simulink model "PI_Controller"  (R2020b)
settings: Solver=VariableStepAuto  StartTime=0.0  StopTime=120  RelTol=1e-3
PostLoadFcn:
  | M=1000;
  | b=50;
  | u=500;
  | 
  | Kp=19.9969;
  | Ki=0.34998;
  | Ts=3.36;
InitFcn:
  | M=1000;
  | b=50;
  | u=500;
  | 
  | Kp=19.9969;
  | Ki=0.34998;
  | Ts=3.36;
settings Model: Creator=home  LastModifiedBy=home
settings DataIOCC: SaveOutput=off  SaveTime=off

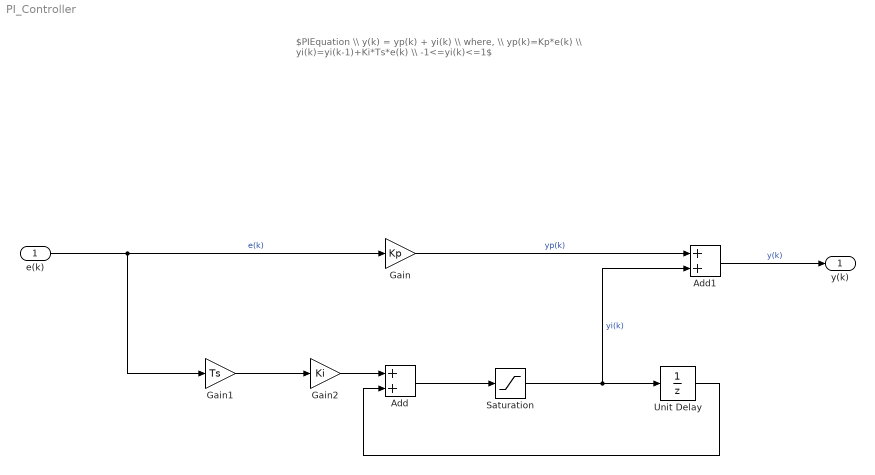
== system PI_Controller ==
  note: $PIEquation \\ y(k) = yp(k) + yi(k) \\ where, \\ yp(k)=Kp*e(k) \\ yi(k)=yi(k-1)+Ki*Ts*e(k) \\ -1<=yi(k)<=1$
  e(k) : Inport  OutDataTypeStr=double  PortDimensions=1  SampleTime=0
  Add : Sum
  Add1 : Sum
  Gain : Gain  Gain=Kp
  Gain1 : Gain  Gain=Ts
  Gain2 : Gain  Gain=Ki
  Saturation : Saturate  UpperLimit=1  LowerLimit=-1
  Unit Delay : UnitDelay  SampleTime=-1  HasFrameUpgradeWarning=on
  y(k) : Outport  OutDataTypeStr=double  PortDimensions=1  SampleTime=0
  wires:
  Add/1 -> Saturation/1
  e(k)/1 -> Gain1/1, Gain/1  "e(k)"
  Add1/1 -> y(k)/1  "y(k)"
  Gain1/1 -> Gain2/1
  Gain2/1 -> Add/1
  Saturation/1 -> Add1/2, Unit Delay/1  "yi(k)"
  Unit Delay/1 -> Add/2
  Gain/1 -> Add1/1  "yp(k)"
